simulink model "Perfect_blend_delayed_Quadcopter_Simulation"  (R2017a)
settings: Solver=ode45  StartTime=0.0  StopTime=35  FixedStep=0.05  MaxStep=0.06  RelTol=1e-3  EnableMultiTasking=on
model workspace (MAT data in the model file):
  MCOS : class17 (value not decoded)
undefined symbols (not defined in the file or in its folder): altitude_error, blend_trigger, current_blend, error1, error2, error3, error4, IC, quadModel
libraries: simulink x4
(part 2 of 2)

== system Perfect_blend_delayed_Quadcopter_Simulation/Quadcopter Dynamics/Motor Dynamics/Throttle To RPM Gain and Cutoff_4 ==
  note: minThr should be a quad.mat value
  note: This gain should be a quad.mat value
  note: This constant should be a quad.mat value
  note: Output equals linearly scaled RPM
      | for given throttle input if throttle input >=Throttle Cuttoff (minThr)
      | else output is zero.
  In5 : Inport
  Constant : Constant  Value=quadModel.b
  Gain : Gain  Gain=quadModel.cr
  Minimum Throttle Cutoff : simulink/Logic and Bit Operations/Compare To Constant  relop=>=  const=quadModel.minThr  OutDataTypeStr=uint8
  Product : Product
  Sum1 : Sum  Inputs=++|
  Out5 : Outport
  wires:
  Minimum Throttle Cutoff/1 -> Product/2
  Product/1 -> Out5/1
  In5/1 -> Gain/1, Minimum Throttle Cutoff/1
  Gain/1 -> Sum1/2
  Sum1/1 -> Product/1
  Constant/1 -> Sum1/1

== matlab function Perfect_blend_delayed_Quadcopter_Simulation/Quadcopter Dynamics/Motor Dynamics/Subsystem/MATLAB Function ==
  data: fault input; nominal_model_input input; rotor_speed output
function rotor_speed = fcn(fault, nominal_model_input)

rotor_speed =(nominal_model_input* (1-fault));

end

== matlab function Perfect_blend_delayed_Quadcopter_Simulation/Attitude Controller/blending  ==
  data: control_signal output; portion input; fault_controller input; nominal_controller input
function control_signal = blending(portion , fault_controller, nominal_controller)

fault_part = (fault_controller * portion);
nominal_portion = 1-portion;
nominal_part = nominal_controller * nominal_portion;
control_signal = fault_part + nominal_part;

end

== matlab function Perfect_blend_delayed_Quadcopter_Simulation/Quadcopter Dynamics/Motor Dynamics/Subsystem1/MATLAB Function ==
  data: fault input; nominal_modal_input input; rotor_speed output
function rotor_speed = fcn(  fault, nominal_modal_input)


rotor_speed =  (nominal_modal_input* (1-fault));

end

== matlab function Perfect_blend_delayed_Quadcopter_Simulation/Position Controller/MATLAB Function ==
  data: y_error input; x_error input; max_error_signal data_store_memory; count data_store_memory; time input; prevTime data_store_memory
function fcn(y_error,x_error,time)
global prevTime;
global max_error_signal;
global count;
%if(abs(y_error) + abs(x_error) > max_error_signal)
if(prevTime+0.1 < time)
    max_error_signal = max_error_signal + abs(y_error) + abs(x_error);
    count =count +1;
    %disp(count);
    prevTime = time;
end
end

== matlab function Perfect_blend_delayed_Quadcopter_Simulation/Quadcopter Dynamics/Motor Dynamics/Subsystem2/MATLAB Function ==
  data: fault input; nominal_modal_input input; rotor_speed output
function rotor_speed = fcn(  fault, nominal_modal_input)


rotor_speed =  (nominal_modal_input* (1-fault));

end

== matlab function Perfect_blend_delayed_Quadcopter_Simulation/Quadcopter Dynamics/Motor Dynamics/Subsystem3/MATLAB Function ==
  data: fault input; nominal_modal_input input; rotor_speed output
function rotor_speed = fcn(  fault, nominal_modal_input)


rotor_speed =  (nominal_modal_input* (1-fault));

end

== matlab function Perfect_blend_delayed_Quadcopter_Simulation/Attitude Controller/blending 1 ==
  data: control_signal output; portion input; fault_controller input; nominal_controller input
function control_signal = blending(portion , fault_controller, nominal_controller)

fault_part = (fault_controller * portion);
nominal_portion = 1-portion;
nominal_part = nominal_controller * nominal_portion;
control_signal = fault_part + nominal_part;

end

== matlab function Perfect_blend_delayed_Quadcopter_Simulation/Attitude Controller/blending 2 ==
  data: control_signal output; portion input; fault_controller input; nominal_controller input
function control_signal = blending(portion , fault_controller, nominal_controller)

fault_part = (fault_controller * portion);
nominal_portion = 1-portion;
nominal_part = nominal_controller * nominal_portion;
control_signal = fault_part + nominal_part;

end

== matlab function Perfect_blend_delayed_Quadcopter_Simulation/Attitude Controller/High Level Randomised Algorithm ==
  data: current_error input; Phi output; Theta output; Psi output; previousTime data_store_memory; blend data_store_memory; time input; Phi_blend data_store_memory; Theta_blend data_store_memory; Psi_blend data_store_memory
function [Phi, Theta, Psi]= fcn(current_error, time)

%global lookup_table;
global previousTime;
%current_error_index = (current_error*1000) +1;
global Phi_blend;
global Theta_blend;
global Psi_blend;

if(previousTime+2 < time)
    if(current_error > 0)
        %stored_value = lookup_table(current_error_index);
        %if( stored_value == -1)
        %generate random blend
        blend = 1;
        Phi = blend;
        Theta= blend;
        Psi = blend;
        
        Phi_blend = blend;
        Theta_blend =blend;
        Psi_blend = blend;
        %   lookup_table(current_error_index) = blend;
        disp(time);
        
        previousTime = time;
    else
        Phi = 0;
        Theta = 0;
        Psi = 0;
        
    end
else
    Phi = Phi_blend;
    Theta= Theta_blend;
    Psi = Psi_blend;
end

== matlab function Perfect_blend_delayed_Quadcopter_Simulation/Position Controller/MATLAB Function1 ==
  data: alt_diff input; y output; altitude_error data_store_memory; time input; PrevTime2 data_store_memory
function y = fcn(alt_diff, time)
global altitude_error;
global PrevTime2;

if(PrevTime2+0.1 < time)
    altitude_error = altitude_error + abs(alt_diff);

    y = altitude_error;
    PrevTime2 = time;
else
    y = altitude_error;
end

== matlab function Perfect_blend_delayed_Quadcopter_Simulation/Attitude Controller/High Level Randomised Algorithm1 ==
  data: x_error input; y_error input; Phi output; Theta output; Psi output; previousTime data_store_memory; blend data_store_memory; time input; Phi_blend data_store_memory; Theta_blend data_store_memory; Psi_blend data_store_memory; rate output; current_error output; rate_of_change data_store_memory; prev_rate_of_change data_store_memory; errors data_store_memory
function [Phi, Theta, Psi, rate, current_error] = fcn(x_error, y_error, time)

%global lookup_table;
global previousTime;
global errors;
%current_error_index = (current_error*1000) +1;
global Phi_blend;
global Theta_blend;
global Psi_blend;
global rate_of_change;
global prev_rate_of_change;

%distance to desired location
current_error = sqrt(x_error^2 + y_error^2);

%previous distance and current distance
if(time > previousTime(5))
    errors(1) = errors(2);
    errors(2) = errors(3);
    errors(3) = errors(4);
    errors(4) = errors(5);
    errors(5) = current_error;

    previousTime(1) = previousTime(2);
    previousTime(2) = previousTime(3);
    previousTime(3) = previousTime(4);
    previousTime(4) = previousTime(5);
    previousTime(5) = time;

    curve = polyfit(previousTime,errors , 4);
    derivative = polyder(curve);
    prev_rate_of_change = rate_of_change;
    rate_of_change =  polyval(derivative,time);
    disp('--------------');
    disp(time);
    disp(rate_of_change);
    disp(abs(current_error));
    rate = rate_of_change;
    
else
    rate = rate_of_change;
end
if(rate_of_change > 0.5 && prev_rate_of_change > 0.5)
%if(current_error > 0.5)
%if(rate_of_change > 1 && current_error > 1)

    blend = rand();
    %blend = 0;
    Phi = blend;
    Theta= blend;
    Psi = blend;
    
    Phi_blend = blend;
    Theta_blend =blend;
    Psi_blend = blend;
    
else
    disp('over');
    Phi = Phi_blend;
    Theta= Theta_blend;
    Psi = Psi_blend;
end
